simulink model "Link_A"  (R2019b)
settings: Solver=FixedStepAuto  StartTime=0  StopTime=15  FixedStep=1  RelTol=1e-3
StopFcn:
  | %set_param(gcb,'TAP_R_INI',[num2str(Tap_pu_R(end)), '  %Updated']);
libraries: simulink x9
(part 2 of 2)

== system Link_A/HVDC Link Steady-State/Converter_Inv/mu_calc_inv ==
  note: Uac_sec_LL_rms / sqrt(2)
  note: pi/6
  note: mu_calc_inv
  note: mu = arcos( cos (gamma - 2 (Xc*3/pi*Id/ Udio)) - gamma
  note: alpha = pi - gamma - mu
  Id : Inport
  gamma : Inport  Port=2
  Udi0 : Inport  Port=3
  Avoid zero : Saturate  UpperLimit=inf  LowerLimit=eps
  Constant : Constant  Value=pi
  Divide1 : Product  Inputs=*/
  Divide2 : Product  Inputs=*/
  Gain2 : Gain  Gain=pi/6
  Min=-1 Max=1 : Saturate  UpperLimit=1  LowerLimit=-1
  Subtract1 : Sum  Inputs=+-
  Subtract2 : Sum  Inputs=+-
  Subtract3 : Sum  Inputs=--+
  Trigonometric Function : Trigonometry  Operator=acos
  Trigonometric Function1 : Trigonometry  Operator=cos
  c : Constant  Value=XC
  mu : Outport
  alpha : Outport  Port=2
  wires:
  Trigonometric Function1/1 -> Subtract1/1
  Subtract3/1 -> alpha/1
  Divide2/1 -> Avoid zero/1  "Is2"
  Gain2/1 -> Divide2/1
  Udi0/1 -> Gain2/1
  Subtract2/1 -> mu/1, Subtract3/1
  gamma/1 -> Trigonometric Function1/1, Subtract3/2, Subtract2/2
  Trigonometric Function/1 -> Subtract2/1
  Subtract1/1 -> Min=-1 Max=1/1
  Divide1/1 -> Subtract1/2
  Avoid zero/1 -> Divide1/2
  Id/1 -> Divide1/1
  c/1 -> Divide2/2
  Min=-1 Max=1/1 -> Trigonometric Function/1
  Constant/1 -> Subtract3/3

== system Link_A/HVDC Link Steady-State/Converter_Rec/P_Q_calc ==
  note: P_Q_calc
  mu : Inport
  Tap_pu : Inport  Port=2
  alpha : Inport  Port=3
  Udio : Inport  Port=4
  "Avoid zero " : Saturate  UpperLimit=inf  LowerLimit=eps
  Gain1 : Gain  Gain=NB
  Gain2 : Gain  Gain=NB
  Id_Iq_Pq_calc : Subsystem
  Terminator : Terminator
  Terminator1 : Terminator
  P : Outport
  Q : Outport  Port=2
  wires:
  Id_Iq_Pq_calc/2(I_q) -> Gain1/1
  Id_Iq_Pq_calc/1(I_d) -> Gain2/1
  alpha/1 -> Id_Iq_Pq_calc/4(angle)
  mu/1 -> Id_Iq_Pq_calc/3(mu)
  Tap_pu/1 -> "Avoid zero "/1
  "Avoid zero "/1 -> Id_Iq_Pq_calc/2(Tap_pu)
  Udio/1 -> Id_Iq_Pq_calc/1(Udio)
  Id_Iq_Pq_calc/3(P_d) -> P/1
  Id_Iq_Pq_calc/4(P_q) -> Q/1
  Gain2/1 -> Terminator/1
  Gain1/1 -> Terminator1/1

== system Link_A/HVDC Link Steady-State/Converter_Rec/Udio_calc ==
  note: VLL_rms
  note: 3*sqrt(2)/pi * Usec_nom/Uprim_nom
  note: Udio_calc
  Eac : Inport
  Tap_pu : Inport  Port=2
  "Avoid zero " : Saturate  UpperLimit=inf  LowerLimit=eps
  Divide3 : Product  Inputs=*/
  k : Gain  Gain=(3*sqrt(2)/pi) * TR
  Udio : Outport
  wires:
  k/1 -> Divide3/1
  Eac/1 -> k/1
  "Avoid zero "/1 -> Divide3/2
  Tap_pu/1 -> "Avoid zero "/1
  Divide3/1 -> Udio/1

== system Link_A/HVDC Link Steady-State/Converter_Rec/alpha_calc_rec ==
  note: Equivalent commtating resistance (Rc)
  note: 3/pi
  note: alpha_calc_rec
  note: Transformer windings resistance drop
  Udio : Inport
  Id : Inport  Port=2
  Ud : Inport  Port=3
  Avoid zero : Saturate  UpperLimit=inf  LowerLimit=eps
  Divide : Product  Inputs=*/
  Gain1 : Gain  Gain=2
  Gain2 : Gain  Gain=3/pi
  Min:-1 Max:1 : Saturate  UpperLimit=1.0  LowerLimit=-1.0
  Product2 : Product  RndMeth=Zero
  Product4 : Product  RndMeth=Zero
  Subtract : Sum  Inputs=+++
  Trigonometric Function1 : Trigonometry  Operator=acos
  c : Constant  Value=XC
  c3 : Constant  Value=RC
  alpha : Outport
  wires:
  c/1 -> Gain2/1
  Id/1 -> Product2/1, Product4/1
  Product2/1 -> Subtract/2  "RcId"
  Gain2/1 -> Product2/2  "Rc"
  Product4/1 -> Subtract/3
  Ud/1 -> Subtract/1
  Subtract/1 -> Divide/1
  Udio/1 -> Avoid zero/1
  Avoid zero/1 -> Divide/2
  Divide/1 -> Min:-1 Max:1/1
  Gain1/1 -> Product4/2
  Trigonometric Function1/1 -> alpha/1
  c3/1 -> Gain1/1
  Min:-1 Max:1/1 -> Trigonometric Function1/1

== system Link_A/HVDC Link Steady-State/Converter_Rec/mu_calc_rec ==
  note: gamma = pi - alpha - mu
  note: mu = arcos( cos (alpha) - 2 (Xc*3/pi*Id/ Udio)) - alpha
  note: mu_calc
  note: pi/6
  note: Uac_sec_LL_rms / sqrt(2)
  Id : Inport
  alpha : Inport  Port=2
  Udi0 : Inport  Port=3
  Avoid zero : Saturate  UpperLimit=inf  LowerLimit=eps
  Constant : Constant  Value=pi
  Divide1 : Product  Inputs=*/
  Divide2 : Product  Inputs=*/
  Gain2 : Gain  Gain=pi/6
  Min=-1 Max=1 : Saturate  UpperLimit=1  LowerLimit=-1
  Subtract1 : Sum  Inputs=+-
  Subtract2 : Sum  Inputs=+-
  Subtract3 : Sum  Inputs=--+
  Trigonometric Function : Trigonometry  Operator=acos
  Trigonometric Function1 : Trigonometry  Operator=cos
  c : Constant  Value=XC
  mu : Outport
  gamma : Outport  Port=2
  wires:
  Constant/1 -> Subtract3/3
  Min=-1 Max=1/1 -> Trigonometric Function/1
  c/1 -> Divide2/2
  Id/1 -> Divide1/1
  Avoid zero/1 -> Divide1/2
  Divide1/1 -> Subtract1/2
  Subtract1/1 -> Min=-1 Max=1/1
  Trigonometric Function/1 -> Subtract2/1
  alpha/1 -> Subtract2/2, Subtract3/2, Trigonometric Function1/1
  Subtract2/1 -> Subtract3/1, mu/1
  Udi0/1 -> Gain2/1
  Gain2/1 -> Divide2/1
  Divide2/1 -> Avoid zero/1  "Is2"
  Subtract3/1 -> gamma/1
  Trigonometric Function1/1 -> Subtract1/1

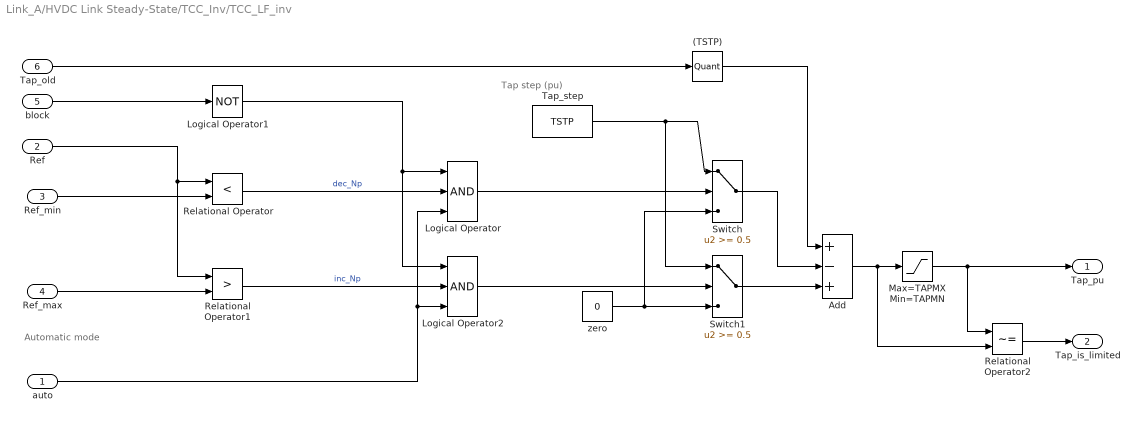
== system Link_A/HVDC Link Steady-State/TCC_Inv/TCC_LF_inv ==
  note: Automatic mode
  note: Tap step (pu)
  auto : Inport
  Ref : Inport  Port=2
  Ref_min : Inport  Port=3
  Ref_max : Inport  Port=4
  block : Inport  Port=5
  Tap_old : Inport  Port=6
  (TSTP) : Quantizer  QuantizationInterval=TSTP
  Add : Sum  Inputs=+-+
  Logical Operator : Logic  Inputs=3  AllPortsSameDT=off  OutDataTypeStr=boolean
  Logical Operator1 : Logic  Operator=NOT  AllPortsSameDT=off  OutDataTypeStr=boolean
  Logical Operator2 : Logic  Inputs=3  AllPortsSameDT=off  OutDataTypeStr=boolean
  Max=TAPMX Min=TAPMN : Saturate  UpperLimit=TAPMX  LowerLimit=TAPMN
  Relational Operator : RelationalOperator  Operator=<  OutDataTypeStr=boolean  RndMeth=Nearest
  Relational Operator1 : RelationalOperator  Operator=>  OutDataTypeStr=boolean  RndMeth=Nearest
  Relational Operator2 : RelationalOperator  Operator=~=  OutDataTypeStr=boolean  RndMeth=Nearest
  Switch : Switch  Threshold=0.5
  Switch1 : Switch  Threshold=0.5
  Tap_step : Constant  Value=TSTP
  zero : Constant  Value=0
  Tap_pu : Outport
  Tap_is_limited : Outport  Port=2
  wires:
  Tap_old/1 -> (TSTP)/1
  (TSTP)/1 -> Add/1
  Ref_min/1 -> Relational Operator/2
  Switch1/1 -> Add/3
  Logical Operator2/1 -> Switch1/2
  Ref/1 -> Relational Operator/1, Relational Operator1/1
  Relational Operator1/1 -> Logical Operator2/2  "inc_Np"
  Relational Operator/1 -> Logical Operator/2  "dec_Np"
  Ref_max/1 -> Relational Operator1/2
  Logical Operator1/1 -> Logical Operator2/1, Logical Operator/1
  block/1 -> Logical Operator1/1
  zero/1 -> Switch/3, Switch1/3
  Tap_step/1 -> Switch/1, Switch1/1
  Add/1 -> Relational Operator2/2, Max=TAPMX Min=TAPMN/1
  auto/1 -> Logical Operator/3, Logical Operator2/3
  Switch/1 -> Add/2
  Max=TAPMX Min=TAPMN/1 -> Relational Operator2/1, Tap_pu/1
  Relational Operator2/1 -> Tap_is_limited/1
  Logical Operator/1 -> Switch/2

== system Link_A/HVDC Link Steady-State/TCC_Rec/TCC_LF ==
  note: Automatic mode
  note: Tap step (pu)
  auto : Inport
  Ref : Inport  Port=2
  Ref_min : Inport  Port=3
  Ref_max : Inport  Port=4
  block : Inport  Port=5
  Tap_old : Inport  Port=6
  (TSTP) : Quantizer  QuantizationInterval=TSTP
  Add : Sum  Inputs=+-+
  Logical Operator : Logic  Inputs=3  AllPortsSameDT=off  OutDataTypeStr=boolean
  Logical Operator1 : Logic  Operator=NOT  AllPortsSameDT=off  OutDataTypeStr=boolean
  Logical Operator2 : Logic  Inputs=3  AllPortsSameDT=off  OutDataTypeStr=boolean
  Max=TAPMX Min=TAPMN : Saturate  UpperLimit=TAPMX  LowerLimit=TAPMN
  Relational Operator : RelationalOperator  Operator=<  OutDataTypeStr=boolean  RndMeth=Nearest
  Relational Operator1 : RelationalOperator  Operator=>  OutDataTypeStr=boolean  RndMeth=Nearest
  Relational Operator2 : RelationalOperator  Operator=~=  OutDataTypeStr=boolean  RndMeth=Nearest
  Switch : Switch  Threshold=0.5
  Switch1 : Switch  Threshold=0.5
  Tap_step : Constant  Value=TSTP
  zero : Constant  Value=0
  Tap_pu : Outport
  Tap_is_limited : Outport  Port=2
  wires:
  Tap_old/1 -> (TSTP)/1
  (TSTP)/1 -> Add/1
  Ref_min/1 -> Relational Operator/2
  Logical Operator/1 -> Switch/2
  Switch1/1 -> Add/3
  Logical Operator2/1 -> Switch1/2
  Ref/1 -> Relational Operator/1, Relational Operator1/1
  Relational Operator1/1 -> Logical Operator2/2  "inc_Np"
  Relational Operator/1 -> Logical Operator/2  "dec_Np"
  Ref_max/1 -> Relational Operator1/2
  Logical Operator1/1 -> Logical Operator/1, Logical Operator2/1
  block/1 -> Logical Operator1/1
  zero/1 -> Switch/3, Switch1/3
  Tap_step/1 -> Switch/1, Switch1/1
  Add/1 -> Relational Operator2/2, Max=TAPMX Min=TAPMN/1
  auto/1 -> Logical Operator/3, Logical Operator2/3
  Switch/1 -> Add/2
  Max=TAPMX Min=TAPMN/1 -> Relational Operator2/1, Tap_pu/1
  Relational Operator2/1 -> Tap_is_limited/1

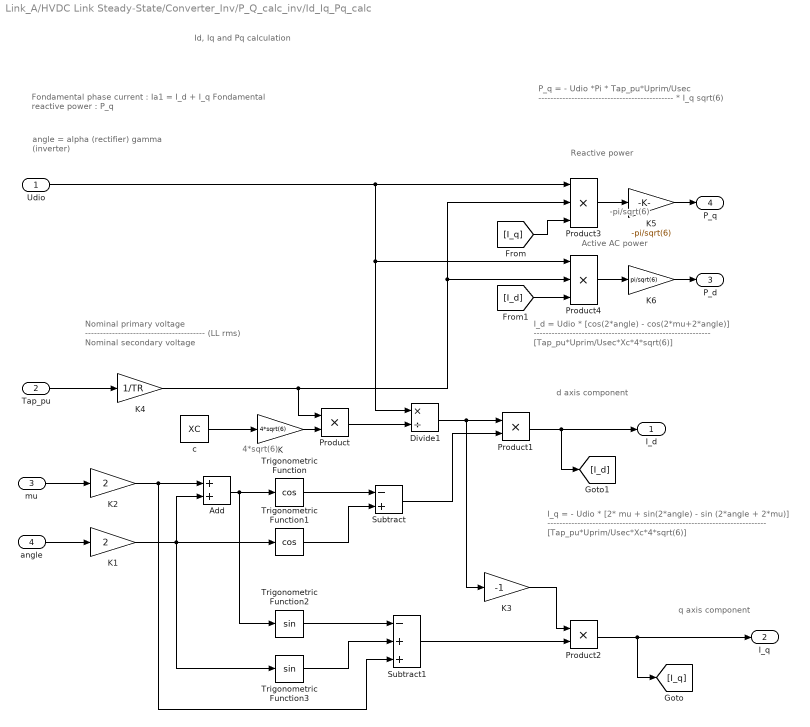
== system Link_A/HVDC Link Steady-State/Converter_Inv/P_Q_calc_inv/Id_Iq_Pq_calc ==
  note: Active AC power
  note: angle = alpha (rectifier)
      |               gamma (inverter)
  note: P_q =  - Udio *Pi * Tap_pu*Uprim/Usec
      |            --------------------------------------------- * I_q
      |                                sqrt(6)
  note: Reactive power
  note: -pi/sqrt(6)
  note: Id, Iq and Pq calculation
  note: q axis component
  note: d axis component
  note: Fondamental phase current :  Ia1 = I_d + I_q
      | Fondamental reactive power : P_q
  note: I_q = - Udio * [2* mu + sin(2*angle) - sin (2*angle + 2*mu)]
      |           -------------------------------------------------------------------------
      |                        [Tap_pu*Uprim/Usec*Xc*4*sqrt(6)]
  note: Nominal primary voltage
      | ----------------------------------------     (LL rms)
      | Nominal secondary voltage
  note: I_d = Udio * [cos(2*angle) - cos(2*mu+2*angle)]
      |           -----------------------------------------------------------
      |                 [Tap_pu*Uprim/Usec*Xc*4*sqrt(6)]
  note: 4*sqrt(6)
  Udio : Inport
  Tap_pu : Inport  Port=2
  mu : Inport  Port=3
  angle : Inport  Port=4
  Add : Sum
  Divide1 : Product  Inputs=*/
  K : Gain  Gain=4*sqrt(6)
  K1 : Gain  Gain=2
  K2 : Gain  Gain=2
  K3 : Gain  Gain=-1
  K4 : Gain  Gain=1/TR
  K5 : Gain  Gain=-pi/sqrt(6)
  K6 : Gain  Gain=pi/sqrt(6)
  Product : Product  RndMeth=Zero
  Product1 : Product  RndMeth=Zero
  Product2 : Product  RndMeth=Zero
  Product3 : Product  Inputs=3  RndMeth=Zero
  Product4 : Product  Inputs=3  RndMeth=Zero
  Subtract : Sum  Inputs=-+
  Subtract1 : Sum  Inputs=-++
  Trigonometric Function : Trigonometry  Operator=cos
  Trigonometric Function1 : Trigonometry  Operator=cos
  Trigonometric Function2 : Trigonometry
  Trigonometric Function3 : Trigonometry
  c : Constant  Value=XC
  I_d : Outport
  I_q : Outport  Port=2
  P_d : Outport  Port=3
  P_q : Outport  Port=4
  wires:
  K6/1 -> P_d/1
  Product4/1 -> K6/1
  [I_d] -> Product4/3
  K5/1 -> P_q/1
  Product3/1 -> K5/1
  K4/1 -> Product4/2, Product3/2, Product/1
  K3/1 -> Product2/1
  c/1 -> K/1
  K/1 -> Product/2
  Product/1 -> Divide1/2
  Udio/1 -> Product4/1, Divide1/1, Product3/1
  Tap_pu/1 -> K4/1
  angle/1 -> K1/1
  K1/1 -> Add/2, Trigonometric Function1/1, Trigonometric Function3/1
  mu/1 -> K2/1
  K2/1 -> Add/1, Subtract1/3
  Add/1 -> Trigonometric Function/1, Trigonometric Function2/1
  Trigonometric Function/1 -> Subtract/1
  Trigonometric Function1/1 -> Subtract/2
  Divide1/1 -> K3/1, Product1/1
  Subtract/1 -> Product1/2
  Product1/1 -> [I_d], I_d/1
  Trigonometric Function2/1 -> Subtract1/1
  Trigonometric Function3/1 -> Subtract1/2
  Subtract1/1 -> Product2/2
  Product2/1 -> [I_q], I_q/1
  [I_q] -> Product3/3

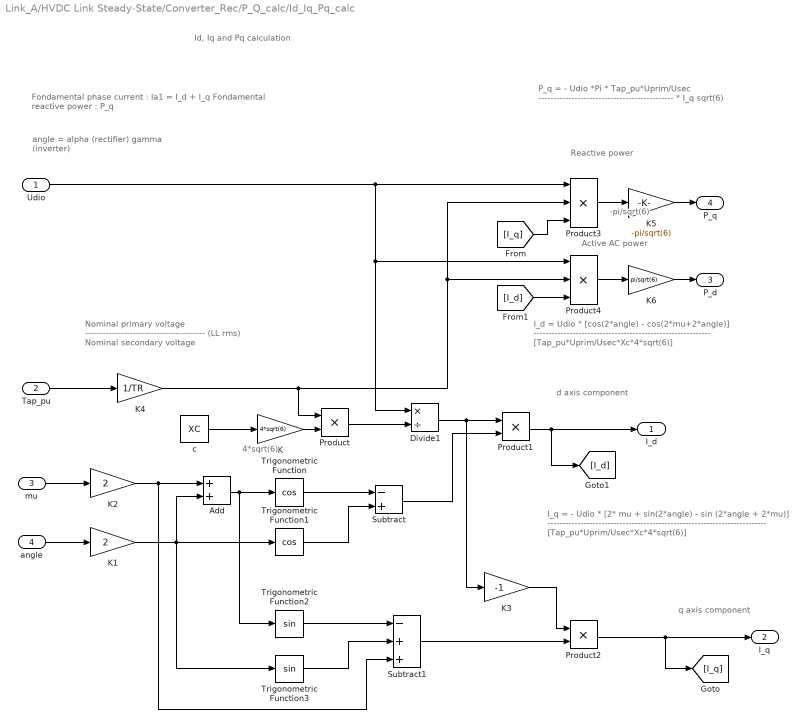
== system Link_A/HVDC Link Steady-State/Converter_Rec/P_Q_calc/Id_Iq_Pq_calc ==
  note: 4*sqrt(6)
  note: I_d = Udio * [cos(2*angle) - cos(2*mu+2*angle)]
      |           -----------------------------------------------------------
      |                 [Tap_pu*Uprim/Usec*Xc*4*sqrt(6)]
  note: Nominal primary voltage
      | ----------------------------------------     (LL rms)
      | Nominal secondary voltage
  note: I_q = - Udio * [2* mu + sin(2*angle) - sin (2*angle + 2*mu)]
      |           -------------------------------------------------------------------------
      |                        [Tap_pu*Uprim/Usec*Xc*4*sqrt(6)]
  note: Fondamental phase current :  Ia1 = I_d + I_q
      | Fondamental reactive power : P_q
  note: d axis component
  note: q axis component
  note: Id, Iq and Pq calculation
  note: -pi/sqrt(6)
  note: Reactive power
  note: P_q =  - Udio *Pi * Tap_pu*Uprim/Usec
      |            --------------------------------------------- * I_q
      |                                sqrt(6)
  note: angle = alpha (rectifier)
      |               gamma (inverter)
  note: Active AC power
  Udio : Inport
  Tap_pu : Inport  Port=2
  mu : Inport  Port=3
  angle : Inport  Port=4
  Add : Sum
  Divide1 : Product  Inputs=*/
  K : Gain  Gain=4*sqrt(6)
  K1 : Gain  Gain=2
  K2 : Gain  Gain=2
  K3 : Gain  Gain=-1
  K4 : Gain  Gain=1/TR
  K5 : Gain  Gain=-pi/sqrt(6)
  K6 : Gain  Gain=pi/sqrt(6)
  Product : Product  RndMeth=Zero
  Product1 : Product  RndMeth=Zero
  Product2 : Product  RndMeth=Zero
  Product3 : Product  Inputs=3  RndMeth=Zero
  Product4 : Product  Inputs=3  RndMeth=Zero
  Subtract : Sum  Inputs=-+
  Subtract1 : Sum  Inputs=-++
  Trigonometric Function : Trigonometry  Operator=cos
  Trigonometric Function1 : Trigonometry  Operator=cos
  Trigonometric Function2 : Trigonometry
  Trigonometric Function3 : Trigonometry
  c : Constant  Value=XC
  I_d : Outport
  I_q : Outport  Port=2
  P_d : Outport  Port=3
  P_q : Outport  Port=4
  wires:
  [I_q] -> Product3/3
  Product2/1 -> [I_q], I_q/1
  Subtract1/1 -> Product2/2
  Trigonometric Function3/1 -> Subtract1/2
  Trigonometric Function2/1 -> Subtract1/1
  Product1/1 -> [I_d], I_d/1
  Subtract/1 -> Product1/2
  Divide1/1 -> Product1/1, K3/1
  Trigonometric Function1/1 -> Subtract/2
  Trigonometric Function/1 -> Subtract/1
  Add/1 -> Trigonometric Function2/1, Trigonometric Function/1
  K2/1 -> Subtract1/3, Add/1
  mu/1 -> K2/1
  K1/1 -> Trigonometric Function3/1, Trigonometric Function1/1, Add/2
  angle/1 -> K1/1
  Tap_pu/1 -> K4/1
  Udio/1 -> Product3/1, Divide1/1, Product4/1
  Product/1 -> Divide1/2
  K/1 -> Product/2
  c/1 -> K/1
  K3/1 -> Product2/1
  K4/1 -> Product/1, Product3/2, Product4/2
  Product3/1 -> K5/1
  K5/1 -> P_q/1
  [I_d] -> Product4/3
  Product4/1 -> K6/1
  K6/1 -> P_d/1
